simulink model "dispatchable_VOC"  (R2022b)
settings: Solver=VariableStepAuto  StartTime=0.0  StopTime=1.5  RelTol=1e-3
InitFcn:
  | R1 = 0.1;
  | L1 = 1e-3;
  | R2 = 0.1;
  | C2 = 50e-6;
  | R3 = 0.1;
  | L3 = 1e-3;
  | Us = 311;
  | D = 10;
  | J = 0.000001;
  | wn = 2*pi*60;
  | 
  | kd = 5;
  | kp = 1;
  | 
  | Ig = 0.1;
  | Bg = 1;
  | Cg = 1;
  | kg = 10;
values from neighbouring files (symbols this model uses):
  C = sqrt(2)/xi/4/V_min_pu^2/(1-V_min_pu^2)    [Init.m]
  C_f = 10e-6    (= 1e-05)    [Init.m]
  iLinit_1 = 0.8    [Init.m]
  Kappa_i = 3*V_nom/S_n    (= 0.2)    [Init.m]
  Kappa_v = V_nom    (= 80)    [Init.m]
  L_f1 = 1.5e-3    (= 0.0015)    [Init.m]
  L_f2 = L_f1    (= 0.0015)    [Init.m]
  PHI = pi/2    (= 1.57079632679)    [Init.m]
  Pref = 000    (= 0)    [Init.m]
  Qref = 000    (= 0)    [Init.m]
  R_f1 = 0.1    [Init.m]
  R_f2 = 0.1    [Init.m]
  Rcf = 0.1    [Init.m]
  V_dc = 250    [Init.m]
  V_grms = 80    [Init.m]
  vCinit_1 = 0.6    [Init.m]
  w_nom = 2*pi*60    (= 376.991118431)    [Init.m]
  xi = 15    [Init.m]
  Xnom = 1    [Init.m]
libraries: spsThreePhaseVIMeasurementLib x3, spsThreePhaseSeriesRLCBranchLib x3, spsGroundLib x2, spsAlphaBetaZerotoabcLib x1, spsDCVoltageSourceLib x1, spsUniversalBridgeLib x1, spsPWMGenerator2LevelLib x1, spsSeriesRLCBranchLib x1, spsThreePhaseProgrammableVoltageSourceLib x1, eePowerMeasurement x1, spsabctoAlphaBetaZeroLib x1, spspowerguiLib x1
settings Model: Creator=得力科技  LastModifiedBy=lumi740
settings SolverCC: AlgebraicLoopSolver=TrustRegion
settings OptimizationCC: LifeSpan=inf
settings DebuggingCC: UnconnectedInputMsg=warning  UnconnectedOutputMsg=warning  UnconnectedLineMsg=warning  SFMachineParentedDataDiag=warning  ArithmeticOperatorsInVariantConditions=warning
settings ModelReferenceCC: EnableRefExpFcnMdlSchedulingChecks=on
settings SFSimCC: CustomCodeUndefinedFunction=UseInterfaceOnly
settings CodeAppCC: StateflowObjectComments=on

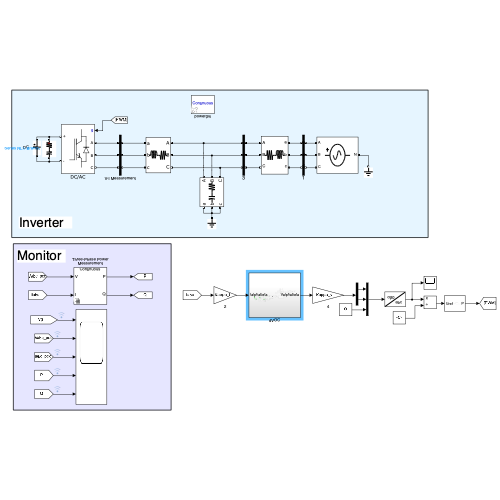
[thumbnail: Simulink's stored preview of the top-level diagram]
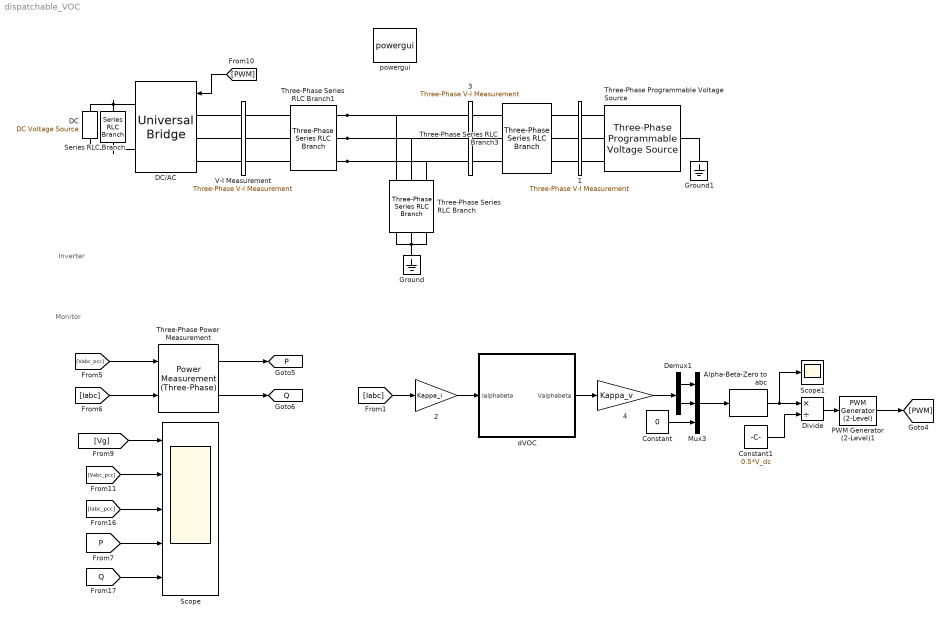
== system dispatchable_VOC ==
  note: Monitor
  note: Inverter
  1 : spsThreePhaseVIMeasurementLib/Three-Phase V-I Measurement  VoltageMeasurement=phase-to-ground  SetLabelV=on  LabelV=Vg  Vpu=off  VpuLL=off  CurrentMeasurement=no  SetLabelI=off  LabelI=Iabc_0  Ipu=off  Pbase=Pnom  Vbase=380  OutputType=Complex  PhasorSimulation=off  PSBequivalent=0
  2 : Gain  Gain=Kappa_i
  3 : spsThreePhaseVIMeasurementLib/Three-Phase V-I Measurement  VoltageMeasurement=phase-to-ground  SetLabelV=on  LabelV=Vabc_pcc  Vpu=off  VpuLL=off  CurrentMeasurement=yes  SetLabelI=on  LabelI=Iabc_pcc  Ipu=off  Pbase=Pnom  Vbase=380  OutputType=Complex  PhasorSimulation=off  PSBequivalent=0
  4 : Gain  Gain=Kappa_v
  Alpha-Beta-Zero to abc : spsAlphaBetaZerotoabcLib/Alpha-Beta-Zero to abc
      settings: LibrarySourceBlock=|
      | sps_lib/Control/Alpha-Beta-Zero
      | to abc
  Constant : Constant  Value=0
  Constant1 : Constant  Value=0.5*V_dc
  "DC " : spsDCVoltageSourceLib/DC Voltage Source  Amplitude=V_dc  Measurements=Voltage
  DC/AC : spsUniversalBridgeLib/Universal Bridge  Arms=3  SnubberResistance=1e5  SnubberCapacitance=inf  Device=IGBT / Diodes  Ron=1e-3  Lon=0  ForwardVoltages="[  0  0  ]"  ForwardVoltage=0  GTOparameters=[ 10e-6 , 20e-6 ]  IGBTparameters=[ 1e-6 , 2e-6 ]  Measurements=None  Measurements_2=None  converterType=Rectifier
  Demux1 : Demux  Outputs=2
  Divide : Product  Inputs=*/
  Ground : spsGroundLib/Ground  LConnTagsString=a
  Ground1 : spsGroundLib/Ground  LConnTagsString=a
  Mux3 : Mux  Inputs=3
  PWM Generator (2-Level)1 : spsPWMGenerator2LevelLib/PWM Generator (2-Level)  ModulatorType=Three-phase bridge (6 pulses)  ModulatorMode=Unsynchronized  Fc=f_sw  Pc=0  nF=27  MinMax="[ -1  1 ]"  SamplingTechnique=Asymmetrical regular (double edge)  ModulatingSignals=off  m=0.8  Freq=60  Phase=0  Ts=0  ShowCarrierOutport=off
  Scope : Scope  NumInputPorts=5
  Scope1 : Scope
  Series RLC Branch : spsSeriesRLCBranchLib/Series RLC Branch  LConnTagsString=__new0  RConnTagsString=__new0  BranchType=RC  Resistance=0.05  Inductance=1e-3  SetiL0=off  InitialCurrent=0  Capacitance=470e-6  Setx0=off  InitialVoltage=0  Measurements=None
  Three-Phase Programmable Voltage Source : spsThreePhaseProgrammableVoltageSourceLib/Three-Phase Programmable Voltage Source  PositiveSequence=[V_grms*sqrt(3) 0 60]  VariationEntity=None  VariationType=Step  VariationTypeAlt=Step  VariationStep=-15  VariationRate=10  VariationMagnitude=0.3  VariationFrequency=2  VariationTiming=[0.4 0.7]  VariationPhaseA=off  Amplitudes=[1 0.8 1.2 1.0]  TimeValues=[0 0.1 0.15 0.2]  HarmonicGeneration=off  HarmonicA=[3 0.2 -25 0]  HarmonicB=[2 0.15 35 2]  Timing="[0.05  3]"  BusType=swing  Pref=0  Qref=0  Qmin=-inf  Qmax=inf
  Three-Phase Series RLC Branch : spsThreePhaseSeriesRLCBranchLib/Three-Phase Series RLC Branch  LConnTagsString=A|B|C  RConnTagsString=A|B|C  BranchType=RC  Resistance=Rcf  Inductance=1e-3  Capacitance=C_f  Measurements=Branch voltages
  Three-Phase Series RLC Branch1 : spsThreePhaseSeriesRLCBranchLib/Three-Phase Series RLC Branch  LConnTagsString=A|B|C  RConnTagsString=A|B|C  BranchType=RL  Resistance=R_f1  Inductance=L_f1  Capacitance=4.5e-3  Measurements=Branch voltages
  Three-Phase Series RLC Branch3 : spsThreePhaseSeriesRLCBranchLib/Three-Phase Series RLC Branch  LConnTagsString=A|B|C  RConnTagsString=A|B|C  BranchType=RL  Resistance=R_f2  Inductance=L_f2  Capacitance=1e-6  Measurements=None
  Three-Phase Power Measurement : eePowerMeasurement/Power Measurement (Three-Phase)  LabelModeActiveChoice=Continuous  F=60  K=[1]  Seq=Positive  Ts=0
  V-I Measurement : spsThreePhaseVIMeasurementLib/Three-Phase V-I Measurement  VoltageMeasurement=phase-to-ground  SetLabelV=on  LabelV=Vabc  Vpu=off  VpuLL=off  CurrentMeasurement=yes  SetLabelI=on  LabelI=Iabc  Ipu=off  Pbase=100e6  Vbase=500e3  OutputType=Complex  PhasorSimulation=off  PSBequivalent=0
  dVOC : Subsystem
  powergui : spspowerguiLib/powergui  Priority=1  SimulationMode=Continuous  SampleTime=5e-6  frequency=60  Iterations=50  frequencyindice=0  Pbase=100e6  ErrMax=1e-4  UnitsV=kV  UnitsW=MW  buscounter=0  FunctionMessages=off  echomessages=off  EnableUseOfTLC=off  CurrentSourceSwitches=off  DisableSnubberDevices=off  DisableRonSwitches=off  DisableVfSwitches=off  DisplayEquations=off  AutomaticDiscreteSolvers=off  SolverType=Tustin  Interpol=off  ExternalGateDelay=off  methode=off  Ts=0  x0status=blocks  SPID=off  SwTol=0  HookPort=off  NonlinearTolerance=1e-4  nMaxIteration=100  ContinueOnMaxIteration=off  RestoreLinks=warning  ResistiveCurrentMeasurement=off  Frange=[0:2:500]  Ylog=off  Xlog=on  ShowGrid=off  save=off  variable=ZData  structure=Ni  ZoomFFT=off  StartTime=0.6  cycles=10  DisplayStyle=1  fundamental=50  FreqAxis=off  MaxFrequency=1000  frequencyindicesteady=1  RmsSteady=1  display=off
  tag scope: P=global, Q=global
  wires:
  [Iabc] -> Three-Phase Power Measurement/2
  [Vabc_pcc] -> Three-Phase Power Measurement/1
  [PWM] -> DC/AC/1
  [Vg] -> Scope/1
  [Iabc_pcc] -> Scope/3
  [P] -> Scope/4
  [Q] -> Scope/5
  Three-Phase Power Measurement/1 -> [P]
  Three-Phase Power Measurement/2 -> [Q]
  [Vabc_pcc] -> Scope/2
  PWM Generator (2-Level)1/1 -> [PWM]
  Alpha-Beta-Zero to abc/1 -> Divide/1, Scope1/1
  [Iabc] -> 2/1
  2/1 -> dVOC/1(Ialphabeta)
  dVOC/1(Valphabeta) -> 4/1
  Demux1/1 -> Mux3/1
  Demux1/2 -> Mux3/2
  Constant/1 -> Mux3/3
  Mux3/1 -> Alpha-Beta-Zero to abc/1
  4/1 -> Demux1/1
  Divide/1 -> PWM Generator (2-Level)1/1
  Constant1/1 -> Divide/2
  connections:
  Three-Phase Series RLC Branch/RConn2 -- Ground/LConn1 -- Three-Phase Series RLC Branch/RConn3 -- Three-Phase Series RLC Branch/RConn1
  Three-Phase Series RLC Branch1/LConn3 -- 3/LConn3 -- Three-Phase Series RLC Branch/LConn3
  Three-Phase Series RLC Branch1/LConn2 -- 3/LConn2 -- Three-Phase Series RLC Branch/LConn2
  Three-Phase Series RLC Branch1/LConn1 -- 3/LConn1 -- Three-Phase Series RLC Branch/LConn1
  1/LConn2 -- Three-Phase Series RLC Branch3/RConn2
  Three-Phase Series RLC Branch3/LConn1 -- 3/RConn1
  Three-Phase Series RLC Branch3/LConn2 -- 3/RConn2
  V-I Measurement/RConn3 -- Three-Phase Series RLC Branch1/RConn3
  DC/AC/RConn1 -- Series RLC Branch/LConn1 -- "DC "/RConn1
  Three-Phase Programmable Voltage Source/RConn2 -- 1/RConn2
  1/LConn1 -- Three-Phase Series RLC Branch3/RConn1
  Three-Phase Programmable Voltage Source/RConn1 -- 1/RConn1
  1/LConn3 -- Three-Phase Series RLC Branch3/RConn3
  Three-Phase Programmable Voltage Source/RConn3 -- 1/RConn3
  Three-Phase Series RLC Branch3/LConn3 -- 3/RConn3
  V-I Measurement/LConn1 -- DC/AC/LConn1
  V-I Measurement/LConn3 -- DC/AC/LConn3
  V-I Measurement/LConn2 -- DC/AC/LConn2
  V-I Measurement/RConn1 -- Three-Phase Series RLC Branch1/RConn1
  V-I Measurement/RConn2 -- Three-Phase Series RLC Branch1/RConn2
  DC/AC/RConn2 -- Series RLC Branch/RConn1 -- "DC "/LConn1
  Three-Phase Programmable Voltage Source/LConn1 -- Ground1/LConn1

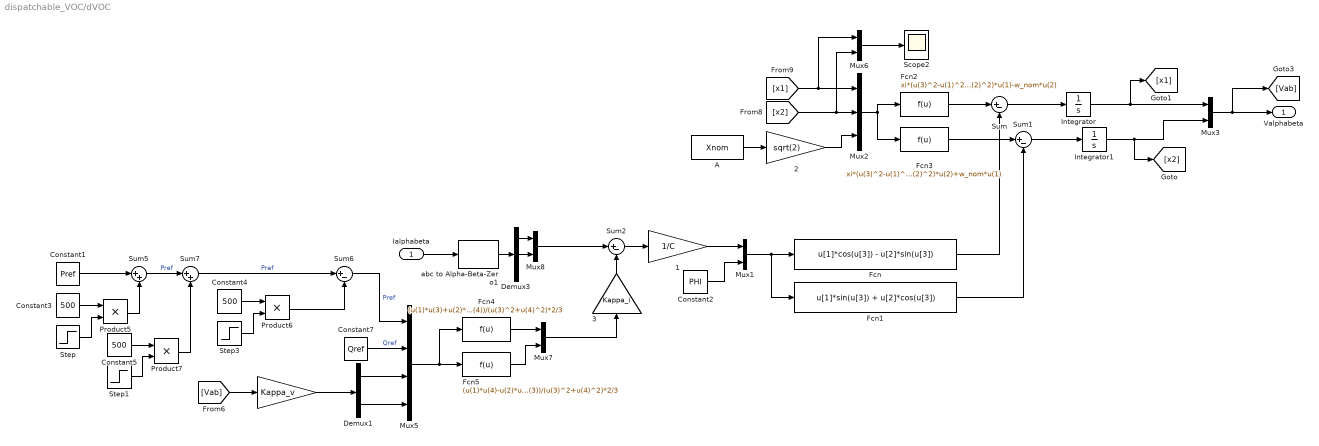
== system dispatchable_VOC/dVOC ==
  Ialphabeta : Inport
  " " : Gain  Gain=Kappa_v
  1 : Gain  Gain=1/C
  2 : Gain  Gain=sqrt(2)
  3 : Gain  Gain=Kappa_i
  A : Constant  Value=Xnom
  Constant1 : Constant  Value=Pref
  Constant2 : Constant  Value=PHI
  Constant3 : Constant  Value=500
  Constant4 : Constant  Value=500
  Constant5 : Constant  Value=500
  Constant7 : Constant  Value=Qref
  Demux1 : Demux  Outputs=2
  Demux3 : Demux  Outputs=3
  Fcn : Fcn  Expr=u[1]*cos(u[3]) - u[2]*sin(u[3])
  Fcn1 : Fcn  Expr=u[1]*sin(u[3]) + u[2]*cos(u[3])
  Fcn2 : Fcn  Expr=xi*(u(3)^2-u(1)^2-u(2)^2)*u(1)-w_nom*u(2)
  Fcn3 : Fcn  Expr=xi*(u(3)^2-u(1)^2-u(2)^2)*u(2)+w_nom*u(1)
  Fcn4 : Fcn  Expr=(u(1)*u(3)+u(2)*u(4))/(u(3)^2+u(4)^2)*2/3
  Fcn5 : Fcn  Expr=(u(1)*u(4)-u(2)*u(3))/(u(3)^2+u(4)^2)*2/3
  Integrator : Integrator  InitialCondition=vCinit_1
  Integrator1 : Integrator  InitialCondition=iLinit_1
  Mux{1,3,6..8} (5 alike) : Mux  Inputs=2
  Mux2 : Mux  Inputs=3
  Mux5 : Mux
  Product5 : Product
  Product6 : Product
  Product7 : Product
  Scope2 : Scope
  Step : Step  Time=0.5  SampleTime=0
  Step1 : Step  Time=0.75  SampleTime=0
  Step3 : Step  SampleTime=0
  Sum{,1..2,6} (4 alike) : Sum  Inputs=|+-
  Sum5 : Sum  Inputs=|++
  Sum7 : Sum  Inputs=|++
  abc to Alpha-Beta-Zero1 : spsabctoAlphaBetaZeroLib/abc to Alpha-Beta-Zero
  Valphabeta : Outport  VectorParamsAs1DForOutWhenUnconnected=off
  wires:
  Fcn5/1 -> Mux7/2
  Constant5/1 -> Product7/1
  Constant4/1 -> Product6/1
  Step/1 -> Product5/2
  Mux6/1 -> Scope2/1
  2/1 -> Mux2/3
  Sum7/1 -> Sum6/1  "Pref"
  Fcn2/1 -> Sum/1
  Step3/1 -> Product6/2
  " "/1 -> Demux1/1
  Product7/1 -> Sum7/2
  [x2] -> Mux6/2, Mux2/2
  Integrator/1 -> Mux3/1, [x1]
  Mux2/1 -> Fcn2/1, Fcn3/1
  3/1 -> Sum2/2
  Fcn3/1 -> Sum1/1
  Product6/1 -> Sum6/2
  Sum6/1 -> Mux5/1  "Pref"
  Step1/1 -> Product7/2
  Constant1/1 -> Sum5/1
  1/1 -> Mux1/1
  Constant3/1 -> Product5/1
  Demux1/2 -> Mux5/4
  Fcn4/1 -> Mux7/1
  Product5/1 -> Sum5/2
  Sum5/1 -> Sum7/1  "Pref"
  Mux1/1 -> Fcn1/1, Fcn/1
  Demux1/1 -> Mux5/3
  Integrator1/1 -> Mux3/2, [x2]
  Sum1/1 -> Integrator1/1
  Sum/1 -> Integrator/1
  Constant2/1 -> Mux1/2
  A/1 -> 2/1
  Sum2/1 -> 1/1
  [x1] -> Mux6/1, Mux2/1
  Constant7/1 -> Mux5/2  "Qref"
  Mux5/1 -> Fcn4/1, Fcn5/1
  [Vab] -> " "/1
  Mux3/1 -> [Vab], Valphabeta/1
  abc to Alpha-Beta-Zero1/1 -> Demux3/1
  Demux3/2 -> Mux8/2
  Demux3/1 -> Mux8/1
  Ialphabeta/1 -> abc to Alpha-Beta-Zero1/1
  Mux8/1 -> Sum2/1
  Fcn/1 -> Sum/2
  Fcn1/1 -> Sum1/2
  Mux7/1 -> 3/1
